simulink model "EstimatorAltitude"  (Simulink 9.1)
settings: Solver=VariableStepAuto  StartTime=0.0  StopTime=10.0  RelTol=1e-3
undefined symbols (not defined in the file): Discrete, Estimator, g, init, Sensors, Time, Ts
libraries: F_Line_block x42, simulink x5, ctrlSharedLib x1, sharedtransform x1
settings Model: LogicAnalyzerSignalOrdering=066e727d-88a7-4005-861a-753b8e9d4f32  Creator=dongw  LastModifiedBy=dongw
settings DataIOCC: SaveFormat=Dataset
settings OptimizationCC: LifeSpan=auto
settings DebuggingCC: UnderspecifiedInitializationDetection=Simplified  MergeDetectMultiDrivingBlocksExec=error  SFUnexpectedBacktrackingDiag=error  SFNoUnconditionalDefaultTransitionDiag=error  SFExecutionAtInitializationDiag=warning
settings HardwareCC: ProdBitPerPointer=64  ProdBitPerSizeT=64  ProdBitPerPtrDiffT=64  ProdLargestAtomicFloat=Float  ProdIntDivRoundTo=Zero  ProdEndianess=LittleEndian  ProdWordSize=64  ProdHWDeviceType=Intel->x86-64 (Windows64)
settings ModelReferenceCC: PropagateSignalLabelsOutOfModel=on
settings CodeAppCC: StateflowObjectComments=off
settings GRTTargetCC: TargetLangStandard=C99 (ISO)  CombineOutputUpdateFcns=on  GRTInterface=off
settings ConfigComp: CovMetricSettings=dwe  CovHtmlReporting=off  CovSaveCumulativeToWorkspaceVar=off  CovSaveSingleToWorkspaceVar=off  CovExternalEMLEnable=on

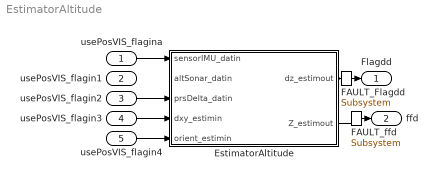
== system EstimatorAltitude ==
  usePosVIS_flagina : Inport
  usePosVIS_flagin1 : Inport  Port=2
  usePosVIS_flagin2 : Inport  Port=3
  usePosVIS_flagin3 : Inport  Port=4
  usePosVIS_flagin4 : Inport  Port=5
  EstimatorAltitude : Subsystem
  Flagdd : Outport
  FAULT_Flagdd : F_Line_block/Subsystem
  ffd : Outport  Port=2
  FAULT_ffd : F_Line_block/Subsystem
  wires:
  usePosVIS_flagina/1 -> EstimatorAltitude/1(sensorIMU_datin)
  usePosVIS_flagin2/1 -> EstimatorAltitude/3(prsDelta_datin)
  usePosVIS_flagin3/1 -> EstimatorAltitude/4(dxy_estimin)
  usePosVIS_flagin4/1 -> EstimatorAltitude/5(orient_estimin)
  EstimatorAltitude/1(dz_estimout) -> FAULT_Flagdd/1
  FAULT_Flagdd/1 -> Flagdd/1
  EstimatorAltitude/2(Z_estimout) -> FAULT_ffd/1
  FAULT_ffd/1 -> ffd/1

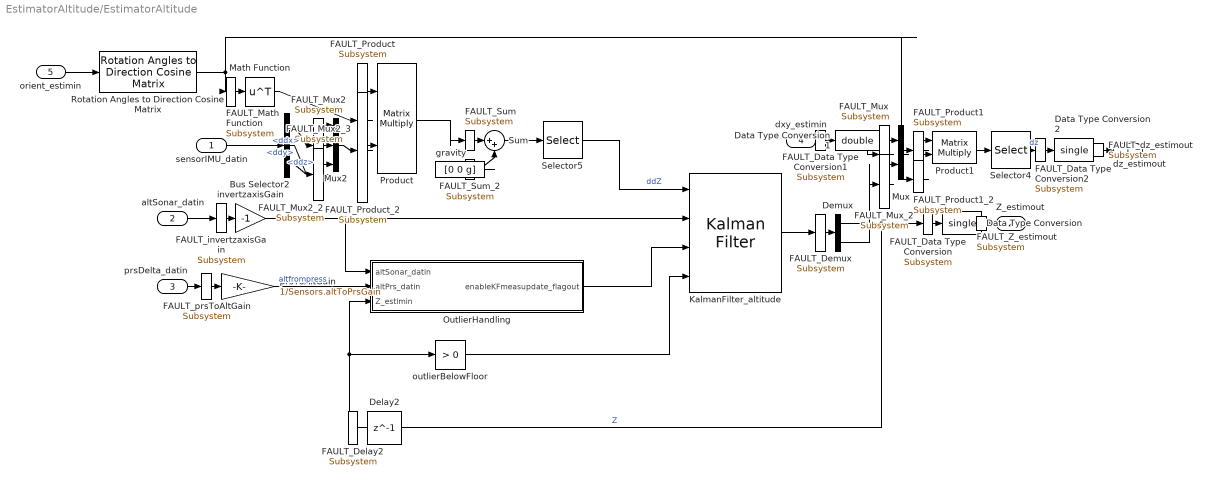
== system EstimatorAltitude/EstimatorAltitude ==
  sensorIMU_datin : Inport
  altSonar_datin : Inport  Port=2
  prsDelta_datin : Inport  Port=3
  dxy_estimin : Inport  Port=4
  orient_estimin : Inport  Port=5
  Bus Selector2 : BusSelector  OutputSignals=ddx,ddy,ddz
  Data Type Conversion : DataTypeConversion  OutDataTypeStr=single  SaturateOnIntegerOverflow=on
  FAULT_Data Type Conversion : F_Line_block/Subsystem
  Data Type Conversion1 : DataTypeConversion  OutDataTypeStr=double  SaturateOnIntegerOverflow=on
  FAULT_Data Type Conversion1 : F_Line_block/Subsystem
  Data Type Conversion2 : DataTypeConversion  OutDataTypeStr=single  SaturateOnIntegerOverflow=on
  FAULT_Data Type Conversion2 : F_Line_block/Subsystem
  Delay2 : Delay  DelayLength=1  InitialCondition=0
  FAULT_Delay2 : F_Line_block/Subsystem
  Demux : Demux  Outputs=2
  FAULT_Demux : F_Line_block/Subsystem
  KalmanFilter_altitude : ctrlSharedLib/Kalman Filter  TimeDomain=Discrete-Time  UseCurrentEstimator=on  ModelSource=Individual A, B, C, D matrices  ModelSourceVariable=sys  A=[1 Ts; 0 1]  B=[0;Ts]  C=[1 0]  D=[0]  NumberOfStates=2  NumberOfInputs=2  NumberOfOutputs=2  InitialEstimateSource=Dialog  X0=[init.posNED(3) 0]  P0=10  UseK=off  UseGH=on  NumberOfProcessNoiseInputs=2  G=Estimator.alt.kf.G  TimeInvariantG=on  H=Estimator.alt.kf.H  TimeInvariantH=on  Q=Estimator.alt.kf.Q  TimeInvariantQ=on  R=Estimator.alt.kf.R  TimeInvariantR=on  N=Estimator.alt.kf.N  TimeInvariantN=on  AddInputPort=on  AddEnablePort=on  ExternalReset=Level hold  OutputEstimatedY=off  OutputP=off  Ts=-1
      settings: SourceProductBaseCode=CT
  Math Function : Math  Operator=transpose  SaturateOnIntegerOverflow=on
  FAULT_Math Function : F_Line_block/Subsystem
  Mux : Mux  Inputs=2
  FAULT_Mux : F_Line_block/Subsystem
  FAULT_Mux_2 : F_Line_block/Subsystem
  Mux2 : Mux  Inputs=3
  FAULT_Mux2 : F_Line_block/Subsystem
  FAULT_Mux2_2 : F_Line_block/Subsystem
  FAULT_Mux2_3 : F_Line_block/Subsystem
  OutlierHandling : Subsystem
  Product : Product  Multiplication=Matrix(*)
  FAULT_Product : F_Line_block/Subsystem
  FAULT_Product_2 : F_Line_block/Subsystem
  Product1 : Product  Multiplication=Matrix(*)
  FAULT_Product1 : F_Line_block/Subsystem
  FAULT_Product1_2 : F_Line_block/Subsystem
  Rotation Angles to Direction Cosine Matrix : sharedtransform/Rotation Angles to Direction Cosine Matrix  rotationOrder=ZYX  aMode=aMode
      settings: SourceProductBaseCode=AE
  Selector4 : Selector  InputPortWidth=3  IndexOptions=Index vector (dialog)  Indices=[3]  OutputSizes=1
  Selector5 : Selector  InputPortWidth=3  IndexOptions=Index vector (dialog)  Indices=[3]  OutputSizes=1
  Sum : Sum  Inputs=|++
  FAULT_Sum : F_Line_block/Subsystem
  FAULT_Sum_2 : F_Line_block/Subsystem
  gravity : Constant  Value=[0 0 g]
  invertzaxisGain : Gain  Gain=-1  ParamDataTypeStr=single  OutDataTypeStr=double
  FAULT_invertzaxisGain : F_Line_block/Subsystem
  outlierBelowFloor : simulink/Logic and Bit Operations/Compare To Constant  relop=>  const=0  OutDataTypeStr=boolean
  prsToAltGain : Gain  Gain=1/Sensors.altToPrsGain
  FAULT_prsToAltGain : F_Line_block/Subsystem
  dz_estimout : Outport
  FAULT_dz_estimout : F_Line_block/Subsystem
  Z_estimout : Outport  Port=2
  FAULT_Z_estimout : F_Line_block/Subsystem
  wires:
  Mux2/1 -> FAULT_Product_2/1
  FAULT_Product_2/1 -> Product/2
  sensorIMU_datin/1 -> Bus Selector2/1
  Bus Selector2/3 -> FAULT_Mux2_3/1  "<ddz>"
  FAULT_Mux2_3/1 -> Mux2/3
  Bus Selector2/2 -> FAULT_Mux2_2/1  "<ddy>"
  FAULT_Mux2_2/1 -> Mux2/2
  Bus Selector2/1 -> FAULT_Mux2/1  "<ddx>"
  FAULT_Mux2/1 -> Mux2/1
  Product1/1 -> Selector4/1
  dxy_estimin/1 -> FAULT_Data Type Conversion1/1
  FAULT_Data Type Conversion1/1 -> Data Type Conversion1/1
  Delay2/1 -> OutlierHandling/3(Z_estimin), outlierBelowFloor/1
  prsToAltGain/1 -> OutlierHandling/2(altPrs_datin)  "altfrompress"
  prsDelta_datin/1 -> FAULT_prsToAltGain/1
  ?FAULT_Add1/1 -> ?Add1/1
  ?FAULT_soonarFilter_IIR/1 -> ?soonarFilter_IIR/1
  FAULT_prsToAltGain/1 -> prsToAltGain/1
  outlierBelowFloor/1 -> KalmanFilter_altitude/4
  Demux/2 -> FAULT_Mux_2/1
  FAULT_Mux_2/1 -> Mux/2
  Selector4/1 -> FAULT_Data Type Conversion2/1  "dz"
  FAULT_Data Type Conversion2/1 -> Data Type Conversion2/1
  Demux/1 -> FAULT_Data Type Conversion/1, FAULT_Delay2/1  "Z"
  FAULT_Data Type Conversion/1 -> Data Type Conversion/1
  FAULT_Delay2/1 -> Delay2/1
  Selector5/1 -> KalmanFilter_altitude/1  "ddZ"
  Mux/1 -> FAULT_Product1_2/1
  FAULT_Product1_2/1 -> Product1/2
  KalmanFilter_altitude/1 -> FAULT_Demux/1
  FAULT_Demux/1 -> Demux/1
  Sum/1 -> Selector5/1
  gravity/1 -> FAULT_Sum_2/1
  FAULT_Sum_2/1 -> Sum/2
  Product/1 -> FAULT_Sum/1
  FAULT_Sum/1 -> Sum/1
  altSonar_datin/1 -> FAULT_invertzaxisGain/1
  FAULT_invertzaxisGain/1 -> invertzaxisGain/1
  orient_estimin/1 -> Rotation Angles to Direction Cosine Matrix/1
  Data Type Conversion/1 -> FAULT_Z_estimout/1
  FAULT_Z_estimout/1 -> Z_estimout/1
  Data Type Conversion1/1 -> FAULT_Mux/1
  FAULT_Mux/1 -> Mux/1
  Math Function/1 -> FAULT_Product/1
  FAULT_Product/1 -> Product/1
  invertzaxisGain/1 -> KalmanFilter_altitude/2, OutlierHandling/1(altSonar_datin)
  Data Type Conversion2/1 -> FAULT_dz_estimout/1
  FAULT_Data Type Conversion/1 -> Data Type Conversion/1
  FAULT_Delay2/1 -> Delay2/1
  FAULT_dz_estimout/1 -> dz_estimout/1
  OutlierHandling/1(enableKFmeasupdate_flagout) -> KalmanFilter_altitude/3
  Rotation Angles to Direction Cosine Matrix/1 -> FAULT_Math Function/1, FAULT_Product1/1
  FAULT_Math Function/1 -> Math Function/1
  FAULT_Product1/1 -> Product1/1

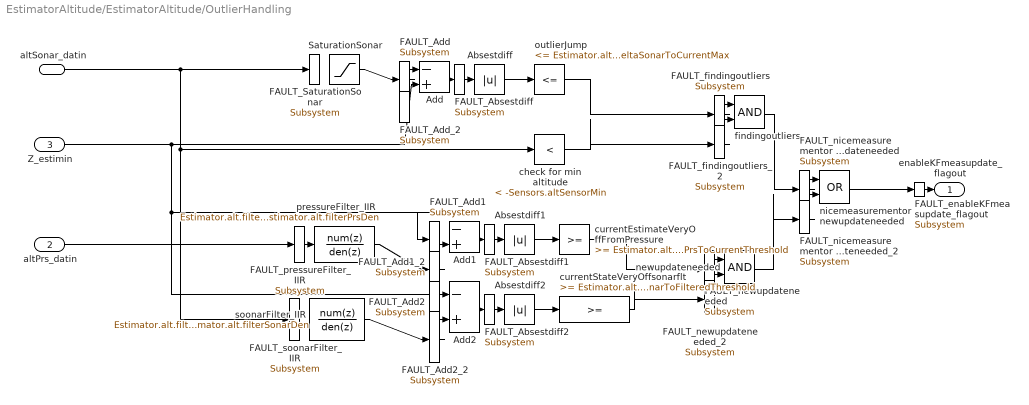
== system EstimatorAltitude/EstimatorAltitude/OutlierHandling ==
  altSonar_datin : Inport
  altPrs_datin : Inport  Port=2
  Z_estimin : Inport  Port=3
  Absestdiff : Abs
  FAULT_Absestdiff : F_Line_block/Subsystem
  Absestdiff1 : Abs
  FAULT_Absestdiff1 : F_Line_block/Subsystem
  Absestdiff2 : Abs
  FAULT_Absestdiff2 : F_Line_block/Subsystem
  Add : Sum  Inputs=-+
  FAULT_Add : F_Line_block/Subsystem
  FAULT_Add_2 : F_Line_block/Subsystem
  Add1 : Sum  Inputs=-+
  FAULT_Add1 : F_Line_block/Subsystem
  FAULT_Add1_2 : F_Line_block/Subsystem
  Add2 : Sum  Inputs=-+
  FAULT_Add2 : F_Line_block/Subsystem
  FAULT_Add2_2 : F_Line_block/Subsystem
  SaturationSonar : Saturate  UpperLimit=-Sensors.altSensorMin  LowerLimit=-inf
  FAULT_SaturationSonar : F_Line_block/Subsystem
  check for min altitude : simulink/Logic and Bit Operations/Compare To Constant  relop=<  const=-Sensors.altSensorMin  OutDataTypeStr=boolean
  currentEstimateVeryOffFromPressure : simulink/Logic and Bit Operations/Compare To Constant  relop=>=  const=Estimator.alt.deltaPrsToCurrentThreshold  OutDataTypeStr=boolean
  currentStateVeryOffsonarflt : simulink/Logic and Bit Operations/Compare To Constant  relop=>=  const=Estimator.alt.deltaSonarToFilteredThreshold  OutDataTypeStr=boolean
  findingoutliers : Logic  AllPortsSameDT=off  OutDataTypeStr=boolean
  FAULT_findingoutliers : F_Line_block/Subsystem
  FAULT_findingoutliers_2 : F_Line_block/Subsystem
  newupdateneeded : Logic  AllPortsSameDT=off  OutDataTypeStr=boolean
  FAULT_newupdateneeded : F_Line_block/Subsystem
  FAULT_newupdateneeded_2 : F_Line_block/Subsystem
  nicemeasurementor newupdateneeded : Logic  Operator=OR  AllPortsSameDT=off  OutDataTypeStr=boolean
  FAULT_nicemeasurementor newupdateneeded : F_Line_block/Subsystem
  FAULT_nicemeasurementor newupdateneeded_2 : F_Line_block/Subsystem
  outlierJump : simulink/Logic and Bit Operations/Compare To Constant  relop=<=  const=Estimator.alt.deltaSonarToCurrentMax  OutDataTypeStr=boolean
  pressureFilter_IIR : DiscreteFilter  Numerator=Estimator.alt.filterPrsNum  Denominator=Estimator.alt.filterPrsDen
  FAULT_pressureFilter_IIR : F_Line_block/Subsystem
  soonarFilter_IIR : DiscreteFilter  Numerator=Estimator.alt.filterSonarNum  Denominator=Estimator.alt.filterSonarDen
  FAULT_soonarFilter_IIR : F_Line_block/Subsystem
  enableKFmeasupdate_flagout : Outport
  FAULT_enableKFmeasupdate_flagout : F_Line_block/Subsystem
  wires:
  Add1/1 -> FAULT_Absestdiff1/1
  FAULT_Absestdiff1/1 -> Absestdiff1/1
  nicemeasurementor newupdateneeded/1 -> FAULT_enableKFmeasupdate_flagout/1
  FAULT_enableKFmeasupdate_flagout/1 -> enableKFmeasupdate_flagout/1
  findingoutliers/1 -> FAULT_nicemeasurementor newupdateneeded/1
  FAULT_nicemeasurementor newupdateneeded/1 -> nicemeasurementor newupdateneeded/1
  check for min altitude/1 -> FAULT_findingoutliers_2/1
  FAULT_findingoutliers_2/1 -> findingoutliers/2
  outlierJump/1 -> FAULT_findingoutliers/1
  FAULT_findingoutliers/1 -> findingoutliers/1
  SaturationSonar/1 -> FAULT_Add/1
  FAULT_Add/1 -> Add/1
  Absestdiff/1 -> outlierJump/1
  Add/1 -> FAULT_Absestdiff/1
  FAULT_Absestdiff/1 -> Absestdiff/1
  newupdateneeded/1 -> FAULT_nicemeasurementor newupdateneeded_2/1
  FAULT_nicemeasurementor newupdateneeded_2/1 -> nicemeasurementor newupdateneeded/2
  Absestdiff2/1 -> currentStateVeryOffsonarflt/1
  altSonar_datin/1 -> FAULT_SaturationSonar/1, FAULT_soonarFilter_IIR/1, check for min altitude/1
  currentEstimateVeryOffFromPressure/1 -> FAULT_newupdateneeded/1
  FAULT_newupdateneeded/1 -> newupdateneeded/1
  Z_estimin/1 -> FAULT_Add1/1, Add2/1, Add/2
  Add2/1 -> FAULT_Absestdiff2/1
  FAULT_Absestdiff2/1 -> Absestdiff2/1
  currentStateVeryOffsonarflt/1 -> FAULT_newupdateneeded_2/1
  FAULT_newupdateneeded_2/1 -> newupdateneeded/2
  pressureFilter_IIR/1 -> FAULT_Add1_2/1
  FAULT_Add1_2/1 -> Add1/2
  altPrs_datin/1 -> FAULT_pressureFilter_IIR/1
  FAULT_pressureFilter_IIR/1 -> pressureFilter_IIR/1
  soonarFilter_IIR/1 -> FAULT_Add2_2/1
  FAULT_Add2_2/1 -> Add2/2
  Absestdiff1/1 -> currentEstimateVeryOffFromPressure/1
